simulink subsystem "Subsystem"  (R2023b)
settings: Solver=VariableStepAuto  StartTime=0.0  StopTime=10.0  RelTol=1e-3
undefined symbols (not defined in the file): designMultirateFIR
libraries: dspmlti4 x4, dspstat3 x3
settings Model: Creator=Fartash  LastModifiedBy=Fartash

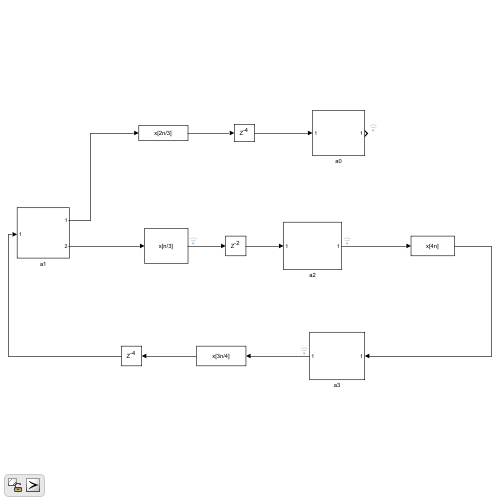
[thumbnail: Simulink's stored preview of the top-level diagram]
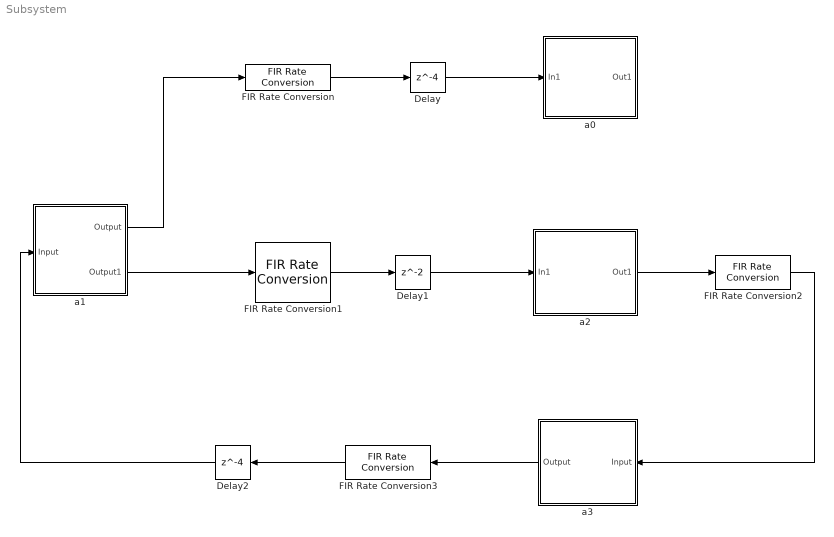
== system Subsystem ==
  Delay : Delay  DelayLength=4
  Delay1 : Delay
  Delay2 : Delay  DelayLength=4
  FIR Rate Conversion : dspmlti4/FIR Rate Conversion  FilterSource=Auto  L=3  h=designMultirateFIR(3,2)  M=2  FilterObject=FRC  rateMode=Enforce single-rate processing  AllowArbitraryInputLength=off  roundingMode=Floor  overflowMode=off  firstCoeffDataTypeStr=Inherit: Same word length as input  firstCoeffMin=[]  firstCoeffMax=[]  firstCoeffLastDataTypeStr=Inherit: Same word length as input  outputDataTypeStr=Inherit: Same as accumulator  outputMin=[]  outputMax=[]  outputLastDataTypeStr=Inherit: Same as accumulator
  FIR Rate Conversion1 : dspmlti4/FIR Rate Conversion  FilterSource=Auto  L=3  h=designMultirateFIR(3,2)  M=1  FilterObject=FRC  rateMode=Enforce single-rate processing  AllowArbitraryInputLength=off  roundingMode=Floor  overflowMode=off  firstCoeffDataTypeStr=Inherit: Same word length as input  firstCoeffMin=[]  firstCoeffMax=[]  firstCoeffLastDataTypeStr=Inherit: Same word length as input  outputDataTypeStr=Inherit: Same as accumulator  outputMin=[]  outputMax=[]  outputLastDataTypeStr=Inherit: Same as accumulator
  FIR Rate Conversion2 : dspmlti4/FIR Rate Conversion  FilterSource=Auto  L=1  h=designMultirateFIR(3,2)  M=4  FilterObject=FRC  rateMode=Enforce single-rate processing  AllowArbitraryInputLength=off  roundingMode=Floor  overflowMode=off  firstCoeffDataTypeStr=Inherit: Same word length as input  firstCoeffMin=[]  firstCoeffMax=[]  firstCoeffLastDataTypeStr=Inherit: Same word length as input  outputDataTypeStr=Inherit: Same as accumulator  outputMin=[]  outputMax=[]  outputLastDataTypeStr=Inherit: Same as accumulator
  FIR Rate Conversion3 : dspmlti4/FIR Rate Conversion  FilterSource=Auto  L=4  h=designMultirateFIR(3,2)  M=3  FilterObject=FRC  rateMode=Enforce single-rate processing  AllowArbitraryInputLength=off  roundingMode=Floor  overflowMode=off  firstCoeffDataTypeStr=Inherit: Same word length as input  firstCoeffMin=[]  firstCoeffMax=[]  firstCoeffLastDataTypeStr=Inherit: Same word length as input  outputDataTypeStr=Inherit: Same as accumulator  outputMin=[]  outputMax=[]  outputLastDataTypeStr=Inherit: Same as accumulator
  a0 : Subsystem
  a1 : Subsystem
  a2 : Subsystem
  a3 : Subsystem
  wires:
  FIR Rate Conversion2/1 -> a3/1(Input)
  a2/1(Out1) -> FIR Rate Conversion2/1
  a3/1(Output) -> FIR Rate Conversion3/1
  FIR Rate Conversion3/1 -> Delay2/1
  FIR Rate Conversion/1 -> Delay/1
  Delay/1 -> a0/1(In1)
  FIR Rate Conversion1/1 -> Delay1/1
  Delay1/1 -> a2/1(In1)
  Delay2/1 -> a1/1(Input)
  a1/1(Output) -> FIR Rate Conversion/1
  a1/2(Output1) -> FIR Rate Conversion1/1

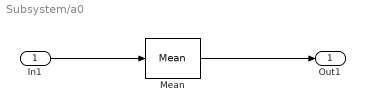
== system Subsystem/a0 ==
  In1 : Inport
  Mean : dspstat3/Mean  run=off  InputProcessing=Columns as channels (frame based)  reset_popup=None  directionMode=Each column  dimension=1  roiEnable=off  roiType=Rectangles  roiPortion=Entire ROI  roiOutput=Individual statistics for each ROI  roiFlag=off  roundingMode=Floor  overflowMode=off  outputDataTypeStr=Inherit: Same as accumulator  outputMin=[]  outputMax=[]  outputLastDataTypeStr=Inherit: Same as accumulator
  Out1 : Outport
  wires:
  Mean/1 -> Out1/1
  In1/1 -> Mean/1

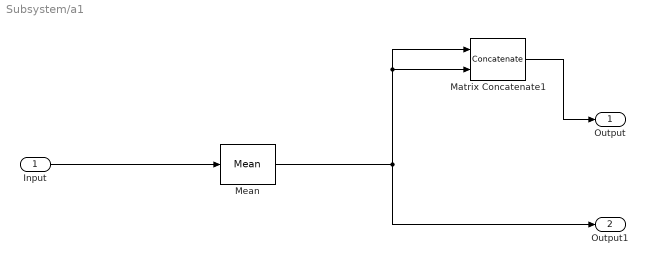
== system Subsystem/a1 ==
  Input : Inport
  Matrix Concatenate1 : Concatenate  ConcatenateDimension=2
  Mean : dspstat3/Mean  run=off  InputProcessing=Columns as channels (frame based)  reset_popup=None  directionMode=Each column  dimension=1  roiEnable=off  roiType=Rectangles  roiPortion=Entire ROI  roiOutput=Individual statistics for each ROI  roiFlag=off  roundingMode=Floor  overflowMode=off  outputDataTypeStr=Inherit: Same as accumulator  outputMin=[]  outputMax=[]  outputLastDataTypeStr=Inherit: Same as accumulator
  Output : Outport
  Output1 : Outport  Port=2
  wires:
  Matrix Concatenate1/1 -> Output/1
  Mean/1 -> Matrix Concatenate1/2, Matrix Concatenate1/1, Output1/1
  Input/1 -> Mean/1

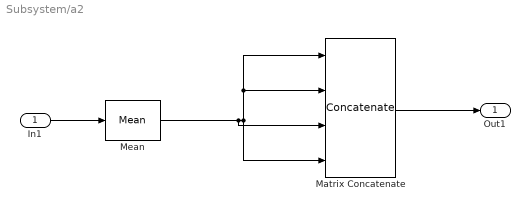
== system Subsystem/a2 ==
  In1 : Inport
  Matrix Concatenate : Concatenate  NumInputs=4  ConcatenateDimension=2
  Mean : dspstat3/Mean  run=off  InputProcessing=Columns as channels (frame based)  reset_popup=None  directionMode=Each column  dimension=1  roiEnable=off  roiType=Rectangles  roiPortion=Entire ROI  roiOutput=Individual statistics for each ROI  roiFlag=off  roundingMode=Floor  overflowMode=off  outputDataTypeStr=Inherit: Same as accumulator  outputMin=[]  outputMax=[]  outputLastDataTypeStr=Inherit: Same as accumulator
  Out1 : Outport
  wires:
  Matrix Concatenate/1 -> Out1/1
  Mean/1 -> Matrix Concatenate/3, Matrix Concatenate/4, Matrix Concatenate/2, Matrix Concatenate/1
  In1/1 -> Mean/1

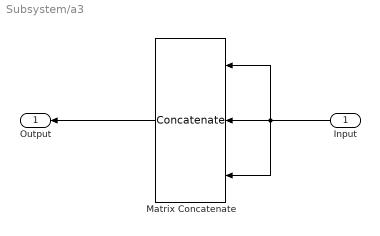
== system Subsystem/a3 ==
  Input : Inport
  Matrix Concatenate : Concatenate  NumInputs=3  ConcatenateDimension=2
  Output : Outport
  wires:
  Matrix Concatenate/1 -> Output/1
  Input/1 -> Matrix Concatenate/2, Matrix Concatenate/3, Matrix Concatenate/1
